simulink model "BoxcarFixedPoint"  (R2021b)
settings: Solver=FixedStepDiscrete  StartTime=0.0  StopTime=0.001  RelTol=1e-3
model workspace (MAT data in the model file):
  test = 0
undefined symbols (not defined in the file): a, b, c
libraries: hdlsllib x4, dspsrcs4 x1
settings Model: DataTypeOverride=Off  FPTShortcutValueString='{{},{''BaselineRun'',1,1,1,''BaselineRun'','''',{},''M'',''F'',''''},{''EmbeddedRun'',1,1,1,''EmbeddedRun'','''',{},''M'','''',''''}}'  Creator=max_d  LastModifiedBy=max_d
settings SolverCC: AlgebraicLoopSolver=TrustRegion  AutoInsertRateTranBlk=on
settings DataIOCC: LimitDataPoints=on  SaveOutput=off  SaveTime=off
settings OptimizationCC: BlockReduction=off  ConditionallyExecuteInputs=off  DefaultParameterBehavior=Inlined  InheritOutputTypeSmallerThanSingle=on  LifeSpan=inf
settings DebuggingCC: SignalRangeChecking=warning  AlgebraicLoopMsg=error  SingleTaskRateTransMsg=error  AllowSymbolicDim=off  StrictBusMsg=ErrorOnBusTreatedAsVector  SFUnexpectedBacktrackingDiag=warning  SFNoUnconditionalDefaultTransitionDiag=warning  SFExecutionAtInitializationDiag=none  SFMachineParentedDataDiag=warning  ArithmeticOperatorsInVariantConditions=warning
settings HardwareCC: ProdBitPerPointer=32  ProdBitPerSizeT=32  ProdBitPerPtrDiffT=32  ProdLargestAtomicFloat=None  ProdIntDivRoundTo=Undefined  ProdEndianess=Unspecified  ProdWordSize=32  ProdHWDeviceType=ASIC/FPGA->ASIC/FPGA  ProdEqTarget=off
settings SFSimCC: SimUseLocalCustomCode=off  CustomCodeUndefinedFunction=UseInterfaceOnly
settings RTWCC: RTWUseLocalCustomCode=off
settings CodeAppCC: StateflowObjectComments=on
settings GRTTargetCC: TargetLangStandard=C89/C90 (ANSI)
settings ConfigComp: CovScope=ReferencedModels  CovMetricSettings=dw  CovSaveCumulativeToWorkspaceVar=on  CovSaveSingleToWorkspaceVar=on  CovExternalEMLEnable=off  CovSFcnEnable=off

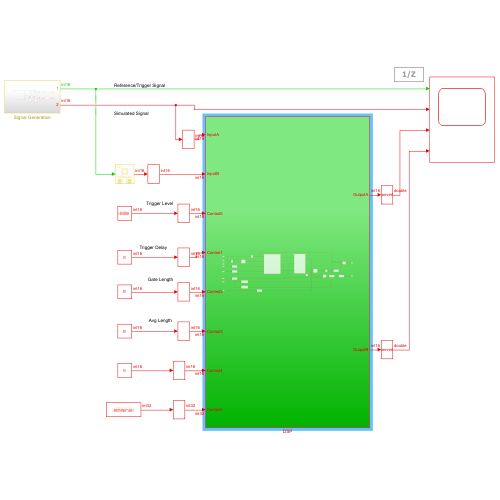
[thumbnail: Simulink's stored preview of the top-level diagram]
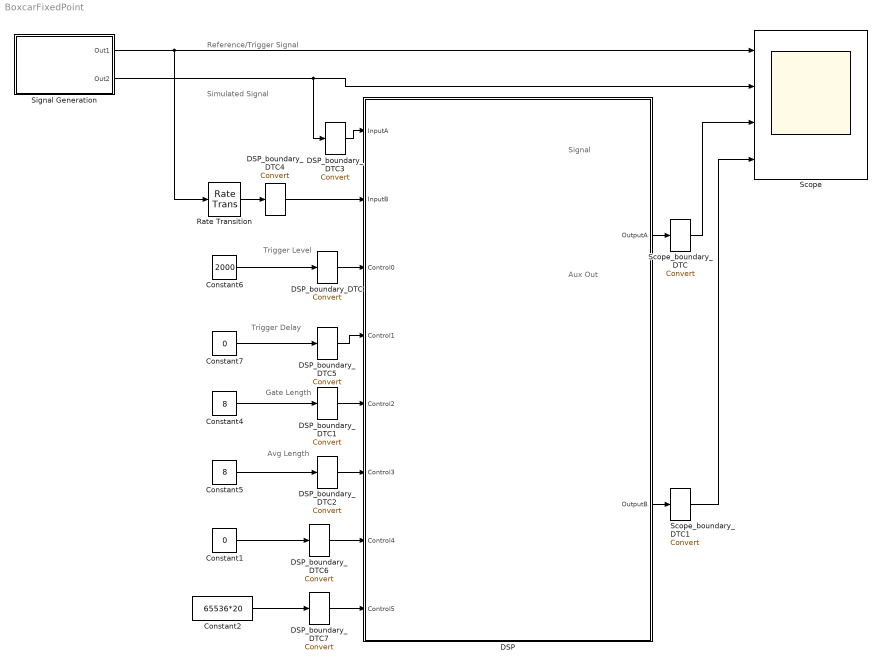
== system BoxcarFixedPoint ==
  note: Reference/Trigger Signal
  note: Simulated Signal
  note: Trigger Level
  note: Trigger Delay
  note: Gate Length
  note: Avg Length
  note: Signal
  note: Aux Out
  Constant1 : Constant  Value=0  OutDataTypeStr=fixdt(1,16,0)  SampleTime=1/312.5e6
  Constant2 : Constant  Value=65536*20  OutDataTypeStr=int32  SampleTime=1/312.5e6
  Constant4 : Constant  Value=8  OutDataTypeStr=fixdt(1,16,0)  SampleTime=1/312.5e6
  Constant5 : Constant  Value=8  OutDataTypeStr=fixdt(1,16,0)  SampleTime=1/312.5e6
  Constant6 : Constant  Value=2000  OutDataTypeStr=fixdt(1,16,0)  SampleTime=1/312.5e6
  Constant7 : Constant  Value=0  OutDataTypeStr=fixdt(1,16,0)  SampleTime=1/312.5e6
  DSP : Subsystem
  DSP_boundary_DTC{,1..7} (8 alike) : DataTypeConversion  SaturateOnIntegerOverflow=on  RndMeth=Zero
  Rate Transition : RateTransition
  Scope : Scope  NumInputPorts=4
  Scope_boundary_DTC : DataTypeConversion  SaturateOnIntegerOverflow=on  RndMeth=Zero
  Scope_boundary_DTC1 : DataTypeConversion  SaturateOnIntegerOverflow=on  RndMeth=Zero
  Signal Generation : Subsystem
  wires:
  Signal Generation/2(Out2) -> Scope/2, DSP_boundary_DTC3/1
  Signal Generation/1(Out1) -> Rate Transition/1, Scope/1
  Constant6/1 -> DSP_boundary_DTC/1
  DSP_boundary_DTC/1 -> DSP/3(Control0)
  Constant4/1 -> DSP_boundary_DTC1/1
  DSP_boundary_DTC1/1 -> DSP/5(Control2)
  Constant5/1 -> DSP_boundary_DTC2/1
  DSP_boundary_DTC2/1 -> DSP/6(Control3)
  DSP_boundary_DTC3/1 -> DSP/1(InputA)
  DSP_boundary_DTC4/1 -> DSP/2(InputB)
  Constant7/1 -> DSP_boundary_DTC5/1
  DSP_boundary_DTC5/1 -> DSP/4(Control1)
  Constant1/1 -> DSP_boundary_DTC6/1
  DSP_boundary_DTC6/1 -> DSP/7(Control4)
  DSP/1(OutputA) -> Scope_boundary_DTC/1
  Scope_boundary_DTC/1 -> Scope/3
  DSP/2(OutputB) -> Scope_boundary_DTC1/1
  Scope_boundary_DTC1/1 -> Scope/4
  Constant2/1 -> DSP_boundary_DTC7/1
  DSP_boundary_DTC7/1 -> DSP/8(Control5)
  Rate Transition/1 -> DSP_boundary_DTC4/1

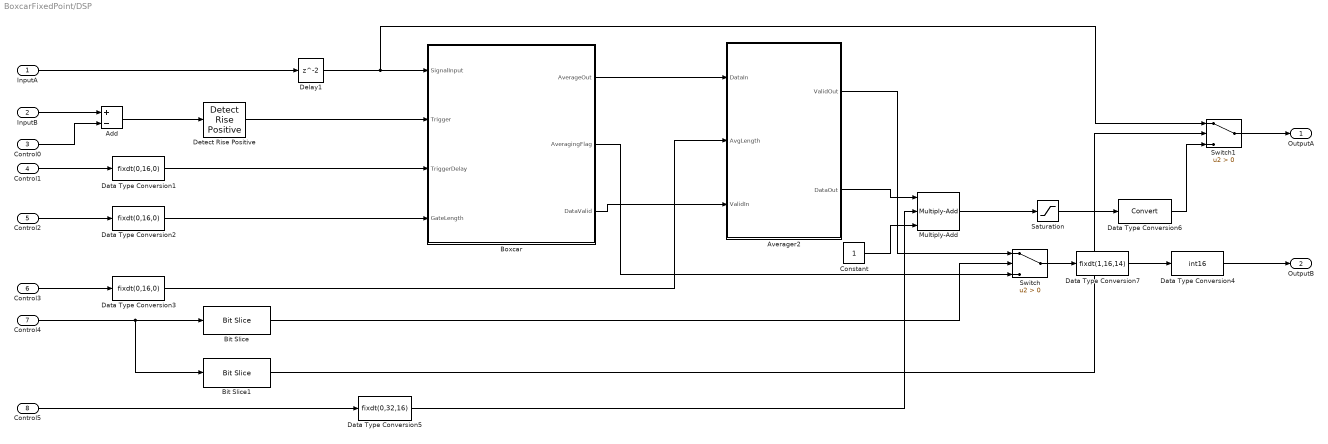
== system BoxcarFixedPoint/DSP ==
  InputA : Inport  OutDataTypeStr=fixdt(1,16,0)
  InputB : Inport  Port=2  OutDataTypeStr=fixdt(1,16,0)
  Control0 : Inport  Port=3  OutDataTypeStr=fixdt(1,16,0)
  Control1 : Inport  Port=4  OutDataTypeStr=fixdt(1,16,0)
  Control2 : Inport  Port=5  OutDataTypeStr=fixdt(1,16,0)
  Control3 : Inport  Port=6  OutDataTypeStr=fixdt(1,16,0)
  Control4 : Inport  Port=7  OutDataTypeStr=fixdt(1,16,0)
  Control5 : Inport  Port=8  OutDataTypeStr=int32
  Add : Sum  Inputs=+-  OutDataTypeStr=fixdt(1,16,0)
  Averager2 : Subsystem  TreatAsAtomicUnit=on  Variant=on  VariantControlMode=label  VariantControl=Choice  LabelModeActiveChoice=(default)
  Bit Slice : hdlsllib/Logic and Bit Operations/Bit Slice  lidx=0  ridx=0
      settings: SourceProductBaseCode=SL
  Bit Slice1 : hdlsllib/Logic and Bit Operations/Bit Slice  lidx=1  ridx=1
      settings: SourceProductBaseCode=SL
  Boxcar : Subsystem  TreatAsAtomicUnit=on  Variant=on  VariantControlMode=label  VariantControl=Choice  LabelModeActiveChoice=(default)
  Constant : Constant  OutDataTypeStr=fixdt(0,1)  SampleTime=1/312.5e6
  Data Type Conversion1 : DataTypeConversion  OutDataTypeStr=fixdt(0,16,0)  ConvertRealWorld=Stored Integer (SI)
  Data Type Conversion2 : DataTypeConversion  OutDataTypeStr=fixdt(0,16,0)  ConvertRealWorld=Stored Integer (SI)
  Data Type Conversion3 : DataTypeConversion  OutDataTypeStr=fixdt(0,16,0)  ConvertRealWorld=Stored Integer (SI)
  Data Type Conversion4 : DataTypeConversion  OutDataTypeStr=int16  ConvertRealWorld=Stored Integer (SI)
  Data Type Conversion5 : DataTypeConversion  OutDataTypeStr=fixdt(0,32,16)  ConvertRealWorld=Stored Integer (SI)
  Data Type Conversion6 : DataTypeConversion
  Data Type Conversion7 : DataTypeConversion  OutDataTypeStr=fixdt(1,16,14)
  Delay1 : Delay  InitialCondition=0
  Detect Rise Positive : hdlsllib/Logic and Bit Operations/Detect Rise Positive  vinit=0  OutDataTypeStr=boolean
      settings: SourceProductBaseCode=SL
  Multiply-Add : hdlsllib/HDL Operations/Multiply-Add  Function=c+(a.*b)  datatype=Inherit: Inherit via internal rule  DoSatur=on  FMA=off
      settings: SourceProductBaseCode=SL
  Saturation : Saturate  UpperLimit=32767  LowerLimit=-32768
  Switch : Switch  Criteria=u2 > Threshold
  Switch1 : Switch  Criteria=u2 > Threshold
  OutputA : Outport  OutDataTypeStr=fixdt(1,16,0)  VectorParamsAs1DForOutWhenUnconnected=off
  OutputB : Outport  Port=2  OutDataTypeStr=fixdt(1,16,0)  VectorParamsAs1DForOutWhenUnconnected=off
  wires:
  InputB/1 -> Add/1
  Control0/1 -> Add/2
  Control3/1 -> Data Type Conversion3/1
  InputA/1 -> Delay1/1
  Switch/1 -> Data Type Conversion7/1
  Control4/1 -> Bit Slice1/1, Bit Slice/1
  Bit Slice/1 -> Switch/2
  Boxcar/2(AveragingFlag) -> Switch/3
  Averager2/1(ValidOut) -> Switch/1
  Delay1/1 -> Switch1/1, Boxcar/1(SignalInput)
  Detect Rise Positive/1 -> Boxcar/2(Trigger)
  Control1/1 -> Data Type Conversion1/1
  Control2/1 -> Data Type Conversion2/1
  Boxcar/1(AverageOut) -> Averager2/1(DataIn)
  Data Type Conversion3/1 -> Averager2/2(AvgLength)
  Boxcar/3(DataValid) -> Averager2/3(ValidIn)
  Data Type Conversion1/1 -> Boxcar/3(TriggerDelay)
  Data Type Conversion2/1 -> Boxcar/4(GateLength)
  Constant/1 -> Multiply-Add/3
  Control5/1 -> Data Type Conversion5/1
  Multiply-Add/1 -> Saturation/1
  Data Type Conversion7/1 -> Data Type Conversion4/1
  Data Type Conversion4/1 -> OutputB/1
  Add/1 -> Detect Rise Positive/1
  Data Type Conversion5/1 -> Multiply-Add/2
  Saturation/1 -> Data Type Conversion6/1
  Switch1/1 -> OutputA/1
  Data Type Conversion6/1 -> Switch1/3
  Bit Slice1/1 -> Switch1/2
  Averager2/2(DataOut) -> Multiply-Add/1

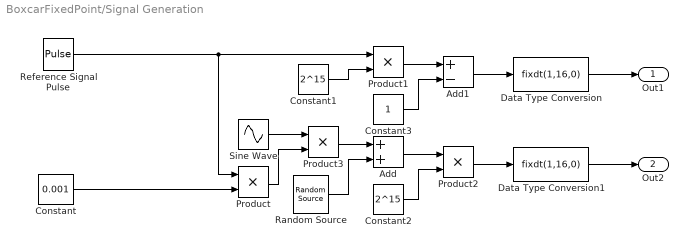
== system BoxcarFixedPoint/Signal Generation ==
  Add : Sum
  Add1 : Sum  Inputs=+-
  Constant : Constant  Value=0.001
  Constant1 : Constant  Value=2^15
  Constant2 : Constant  Value=2^15
  Constant3 : Constant
  Data Type Conversion : DataTypeConversion  OutDataTypeStr=fixdt(1,16,0)
  Data Type Conversion1 : DataTypeConversion  OutDataTypeStr=fixdt(1,16,0)
  Product{,1..3} (4 alike) : Product
  Random Source : dspsrcs4/Random Source  SrcType=Uniform  NormMethod=Ziggurat  CltLength=12  MinVal=-0.001  MaxVal=0.001  MeanVal=0  VarVal=1  RepMode=Not repeatable  rawSeed=1  IsInherit=off  SampMode=Discrete  SampTime=1/312.5e6  SampFrame=1  DataType=Double  OutComplex=Real  OutputFrames=off
  Reference Signal Pulse : DiscretePulseGenerator  PulseType=Time based  Period=100/(312.5e6)  PulseWidth=16
  Sine Wave : Sin  Amplitude=0.5  Bias=0.5  Frequency=2*pi*10e3  SampleTime=1/312.5e6
  Out1 : Outport  OutDataTypeStr=int16
  Out2 : Outport  Port=2  OutDataTypeStr=int16
  wires:
  Data Type Conversion/1 -> Out1/1
  Reference Signal Pulse/1 -> Product/1, Product1/1
  Constant3/1 -> Add1/2
  Add1/1 -> Data Type Conversion/1
  Product1/1 -> Add1/1
  Product3/1 -> Add/1
  Random Source/1 -> Add/2
  Add/1 -> Product2/1
  Sine Wave/1 -> Product3/1
  Product2/1 -> Data Type Conversion1/1
  Constant2/1 -> Product2/2
  Constant/1 -> Product/2
  Product/1 -> Product3/2
  Constant1/1 -> Product1/2
  Data Type Conversion1/1 -> Out2/1

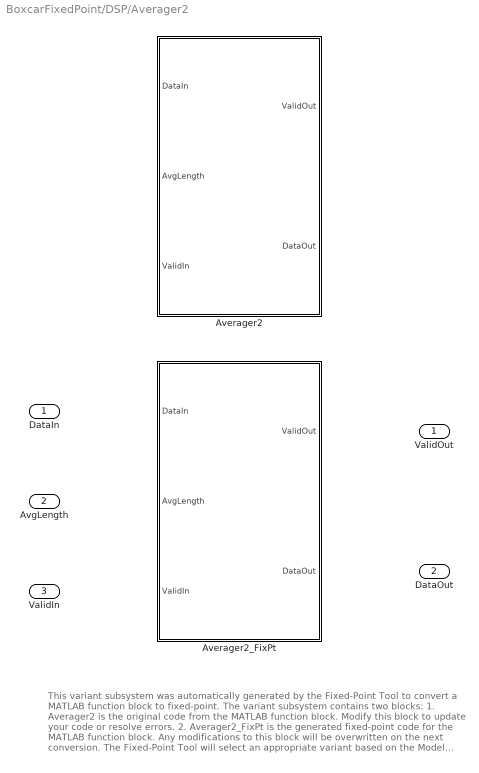
== system BoxcarFixedPoint/DSP/Averager2 ==
  note: This variant subsystem was automatically generated by the Fixed-Point Tool to convert a MATLAB function block to fixed-point.
      |
      | The variant subsystem contains two blocks:
      | 1. Averager2 is the original code from the MATLAB function block. Modify this block to update your code or resolve errors.
      |
      | 2. Averager2_FixPt is the generated fixed-point code for the MATLAB function block. Any modifications to this block will be overwritten on the next conversion.
      |
      | The Fixed-Point Tool will select an appropriate variant based on the Model Settings. Learn more. .
  DataIn : Inport
  AvgLength : Inport  Port=2
  ValidIn : Inport  Port=3
  Averager2 : MATLAB Function  TreatAsAtomicUnit=on  VariantControl=false()
  Averager2_FixPt : MATLAB Function  TreatAsAtomicUnit=on  VariantControl=(default)
  ValidOut : Outport
  DataOut : Outport  Port=2

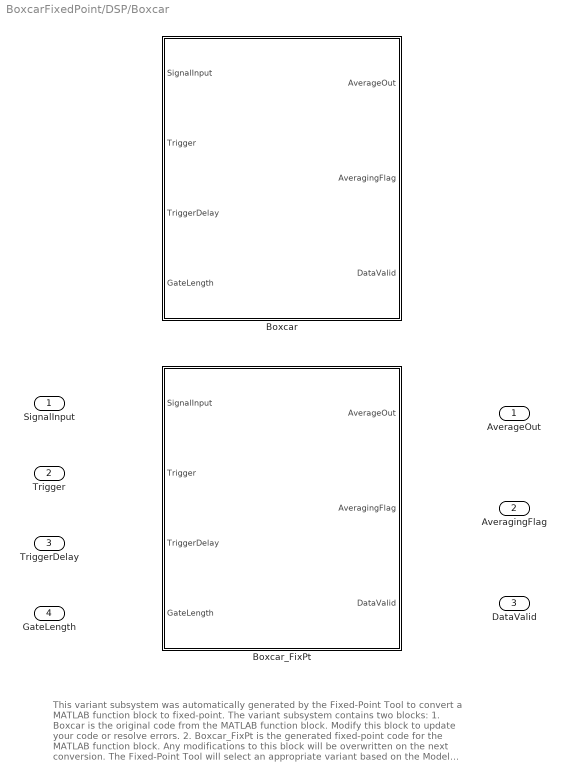
== system BoxcarFixedPoint/DSP/Boxcar ==
  note: This variant subsystem was automatically generated by the Fixed-Point Tool to convert a MATLAB function block to fixed-point.
      |
      | The variant subsystem contains two blocks:
      | 1. Boxcar is the original code from the MATLAB function block. Modify this block to update your code or resolve errors.
      |
      | 2. Boxcar_FixPt is the generated fixed-point code for the MATLAB function block. Any modifications to this block will be overwritten on the next conversion.
      |
      | The Fixed-Point Tool will select an appropriate variant based on the Model Settings. Learn more. .
  SignalInput : Inport
  Trigger : Inport  Port=2
  TriggerDelay : Inport  Port=3
  GateLength : Inport  Port=4
  Boxcar : MATLAB Function  TreatAsAtomicUnit=on  VariantControl=false()
  Boxcar_FixPt : MATLAB Function  TreatAsAtomicUnit=on  VariantControl=(default)
  AverageOut : Outport
  AveragingFlag : Outport  Port=2
  DataValid : Outport  Port=3

== matlab function BoxcarFixedPoint/DSP/Boxcar/Boxcar ==
  data: SignalInput input; AverageOut output; Trigger input; TriggerDelay input; GateLength input; AveragingFlag output; DataValid output
function [AverageOut,AveragingFlag,DataValid] = Boxcar(SignalInput, Trigger, TriggerDelay, GateLength)

persistent AvgOut;
if isempty(AvgOut)
    AvgOut = 0;
end


persistent cnt1;
if isempty(cnt1)
    cnt1 = 0;
end

persistent cnt2;
if isempty(cnt2)
    cnt2 = 0;
end


persistent AvgFlag;
if isempty(AvgFlag)
    AvgFlag = 0;
end

persistent DValid;
if isempty(DValid)
    DValid = 0;
end

S1 = 0; %Waiting for trigger
S2 = 1;
S3 = 2;

persistent current_state;
if isempty(current_state)
    current_state = S1;   
end

switch(current_state)

    case S1
        DValid = 0;


        if Trigger == 1
            current_state = S2;
            cnt1 = TriggerDelay;
        else
            current_state = S1;
        end

    case S2

        if cnt1 == 0
            current_state = S3;
            cnt2 = GateLength;
            AvgOut = 0;
        else
            cnt1 = cnt1-1;
        end

    case S3

        if cnt2 == 0
            current_state = S1;
            DValid = 0;
        else
            AvgOut = AvgOut + SignalInput;
            AvgFlag = 1;
            cnt2 = cnt2-1;
            if cnt2 == 0
                DValid = 1;
                AvgFlag = 0;
            end
        end
end

AverageOut = AvgOut;
DataValid = DValid;
AveragingFlag = AvgFlag;



end

== matlab function BoxcarFixedPoint/DSP/Boxcar/Boxcar_FixPt ==
  settings: fimath=fimath('RoundingMethod', 'Floor', 'OverflowAction', 'Wrap', 'ProductMode', 'FullPrecision', 'MaxProductWordLength', 128, 'SumMode', 'FullPrecision', 'MaxSumWordLength', 128)
  data: SignalInput input; AverageOut output; Trigger input; TriggerDelay input; GateLength input; AveragingFlag output; DataValid output
%auto-generated
%#codegen
function [AverageOut,AveragingFlag,DataValid] = Boxcar_fixpt(SignalInput, Trigger, TriggerDelay, GateLength)

fm = get_fimath();
GateLength = fi(GateLength, 0, 16, 0, fm);
SignalInput = fi(SignalInput, 1, 16, 0, fm);
TriggerDelay = fi(TriggerDelay, 0, 16, 0, fm);

persistent AvgOut;
if isempty(AvgOut)
    AvgOut = fi(0, 1, 32, 0, fm);
end


persistent cnt1;
if isempty(cnt1)
    cnt1 = fi(0, 0, 16, 0, fm);
end

persistent cnt2;
if isempty(cnt2)
    cnt2 = fi(0, 0, 16, 0, fm);
end


persistent AvgFlag;
if isempty(AvgFlag)
    AvgFlag = fi(0, 0, 1, 0, fm);
end

persistent DValid;
if isempty(DValid)
    DValid = fi(0, 0, 1, 0, fm);
end

S1 = fi(0, 0, 2, 0, fm); %Waiting for trigger
S2 = fi(1, 0, 2, 0, fm);
S3 = fi(2, 0, 2, 0, fm);

persistent current_state;
if isempty(current_state)
    current_state = fi(S1, 0, 2, 0, fm);   
end

switch(current_state)

    case S1
        DValid(:) = 0;


        if Trigger == 1
            current_state(:) = S2;
            cnt1(:) = TriggerDelay;
        else
            current_state(:) = S1;
        end

    case S2

        if cnt1 == fi(0, 0, 1, 0, fm)
            current_state(:) = S3;
            cnt2(:) = GateLength;
            AvgOut(:) = 0;
        else
            cnt1(:) = fi_signed(cnt1)-fi(1, 0, 1, 0, fm);
        end

    case S3

        if cnt2 == fi(0, 0, 1, 0, fm)
            current_state(:) = S1;
            DValid(:) = 0;
        else
            AvgOut(:) = AvgOut + SignalInput;
            AvgFlag(:) = 1;
            cnt2(:) = fi_signed(cnt2)-fi(1, 0, 1, 0, fm);
            if cnt2 == fi(0, 0, 1, 0, fm)
                DValid(:) = 1;
                AvgFlag(:) = 0;
            end
        end
end

AverageOut = fi(AvgOut, 1, 32, 0, fm);
DataValid = fi(DValid, 0, 1, 0, fm);
AveragingFlag = fi(AvgFlag, 0, 1, 0, fm);



end



function y = fi_signed(a)
    coder.inline( 'always' );
    if isfi( a ) && ~(issigned( a ))
        nt = numerictype( a );
        new_nt = numerictype( 1, nt.WordLength + 1, nt.FractionLength );
        y = fi( a, new_nt, fimath( a ) );
    else
        y = a;
    end
end

function fm = get_fimath()
	fm = fimath('RoundingMethod', 'Floor',...
	     'OverflowAction', 'Wrap',...
	     'ProductMode','FullPrecision',...
	     'MaxProductWordLength', 128,...
	     'SumMode','FullPrecision',...
	     'MaxSumWordLength', 128);
end

== matlab function BoxcarFixedPoint/DSP/Averager2/Averager2_FixPt ==
  settings: fimath=fimath('RoundingMethod', 'Floor', 'OverflowAction', 'Wrap', 'ProductMode', 'FullPrecision', 'MaxProductWordLength', 128, 'SumMode', 'FullPrecision', 'MaxSumWordLength', 128)
  data: DataIn input; AvgLength input; ValidIn input; ValidOut output; DataOut output
%auto-generated
function [ValidOut,DataOut] = Average_fixpt(DataIn,AvgLength,ValidIn)
%#codegen

fm = get_fimath();
AvgLength = fi(AvgLength, 0, 16, 0, fm);
DataIn = fi(DataIn, 1, 32, 0, fm);
ValidIn = fi(ValidIn, 0, 1, 0, fm);

persistent AvgOut;
if isempty(AvgOut)
    AvgOut = fi(0, 1, 48, 0, fm);
end

persistent DataOutReg;
if isempty(DataOutReg)
    DataOutReg = fi(0, 1, 48, 0, fm);
end

persistent ValidOutReg;
if isempty(ValidOutReg)
    ValidOutReg = fi(0, 0, 1, 0, fm);
end

persistent cnt1;
if isempty(cnt1)
    cnt1 = fi(0, 0, 16, 0, fm);
end


S1 = fi(0, 0, 1, 0, fm); %Waiting for trigger
S2 = fi(1, 0, 1, 0, fm);

persistent current_state;
if isempty(current_state)
    current_state = fi(S1, 0, 1, 0, fm);   
end

switch(current_state)

    case S1

        if ValidIn == fi(1, 0, 1, 0, fm)
            current_state(:) = S2;
            cnt1(:) = fi_signed(AvgLength)-fi(1, 0, 1, 0, fm);
            AvgOut(:) = DataIn;
        else
            current_state(:) = S1;
        end

    case S2

%         if cnt1 == 0
%             current_state = S1;
%             AvgOut = 0;
%         else
            if ValidIn == fi(1, 0, 1, 0, fm)
                AvgOut(:) = AvgOut+DataIn;
                cnt1(:) = fi_signed(cnt1)-fi(1, 0, 1, 0, fm);
            end
            if cnt1 == fi(0, 0, 1, 0, fm)
                DataOutReg(:) = AvgOut;
                ValidOutReg(:) = 1;
                current_state(:) = S1;
            end
        %end



end

DataOut = fi(DataOutReg, 1, 48, 0, fm);
ValidOut = fi(ValidOutReg, 0, 1, 0, fm);

end



function y = fi_signed(a)
    coder.inline( 'always' );
    if isfi( a ) && ~(issigned( a ))
        nt = numerictype( a );
        new_nt = numerictype( 1, nt.WordLength + 1, nt.FractionLength );
        y = fi( a, new_nt, fimath( a ) );
    else
        y = a;
    end
end

function fm = get_fimath()
	fm = fimath('RoundingMethod', 'Floor',...
	     'OverflowAction', 'Wrap',...
	     'ProductMode','FullPrecision',...
	     'MaxProductWordLength', 128,...
	     'SumMode','FullPrecision',...
	     'MaxSumWordLength', 128);
end

== matlab function BoxcarFixedPoint/DSP/Averager2/Averager2 ==
  data: DataIn input; AvgLength input; ValidIn input; ValidOut output; DataOut output
function [ValidOut,DataOut] = Average(DataIn,AvgLength,ValidIn)
%#codegen

persistent AvgOut;
if isempty(AvgOut)
    AvgOut = 0;
end

persistent DataOutReg;
if isempty(DataOutReg)
    DataOutReg = 0;
end

persistent ValidOutReg;
if isempty(ValidOutReg)
    ValidOutReg = 0;
end

persistent cnt1;
if isempty(cnt1)
    cnt1 = 0;
end


S1 = 0; %Waiting for trigger
S2 = 1;

persistent current_state;
if isempty(current_state)
    current_state = S1;   
end

switch(current_state)

    case S1

        if ValidIn == 1
            current_state = S2;
            cnt1 = AvgLength-1;
            AvgOut = DataIn;
        else
            current_state = S1;
        end

    case S2

%         if cnt1 == 0
%             current_state = S1;
%             AvgOut = 0;
%         else
            if ValidIn == 1
                AvgOut = AvgOut+DataIn;
                cnt1 = cnt1-1;
            end
            if cnt1 == 0
                DataOutReg = AvgOut;
                ValidOutReg = 1;
                current_state = S1;
            end
        %end



end

DataOut = DataOutReg;
ValidOut = ValidOutReg;

end
